simulink model "Test_N7"  (R2020b)
settings: Solver=ode3  StartTime=0.0  StopTime=inf  FixedStep=0.05  RelTol=1e-3
libraries: XBotBlockToolbox x2, Utilities x1

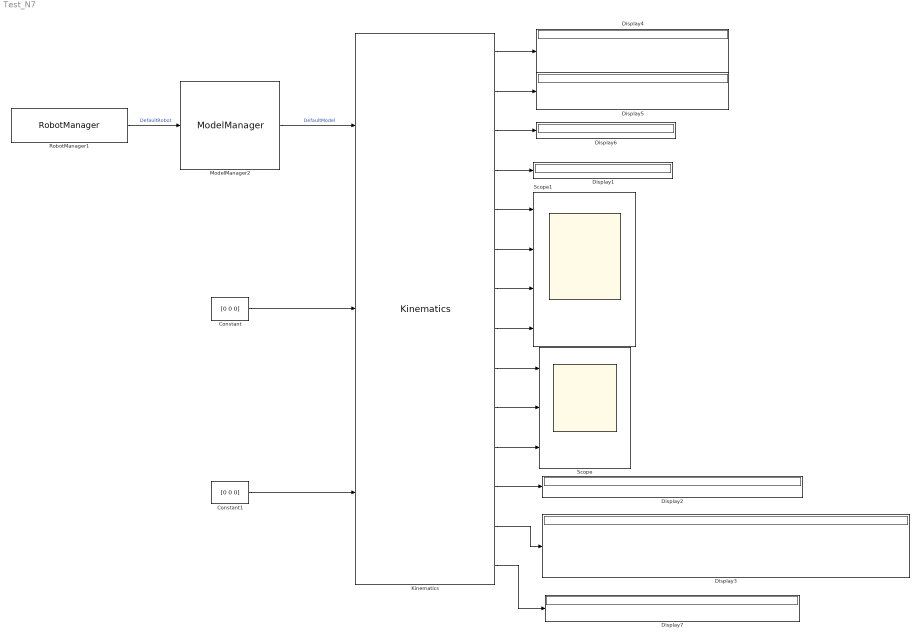
== system Test_N7 ==
  Constant : Constant  Value=[0 0 0]
  Constant1 : Constant  Value=[0 0 0]
  Display{1..7} (7 alike) : Display
  Kinematics : Utilities/Kinematics  ModelName=DefaultModel  PoseList={ 'Pose', 'RotMatrix', 'PointPos', 'PointAcc' }  SourceFrame=LWrMot3  LinkNamePose=LWrMot3  TwistList={ 'v_tw', 'a_tw', 'v_tw_rel', 'a_tw_rel' }  LinkName=LWrMot3  BaseLinkName=base_link  COMList={ 'p_COM', 'v_COM', 'a_COM', 'CM', 'CM_Matrix', 'CMMdotQdot' }
  ModelManager2 : XBotBlockToolbox/ModelManager  ModelName=DefaultModel  RobotName=DefaultRobot  UseExtModel=Off  SyncWithRobot=On  GetFloatingBaseList={}  SetFloatingBaseComponent=Off  GravityRequest=Off  ReadingsList={}  MechanicalLimitsList={}  MechanicalLimitsCheck=Off  MechanicalLimitsEnforce=Off  SensorList={}  ReferencesList={}  OldModelName=DefaultModel
  RobotManager1 : XBotBlockToolbox/RobotManager  RobotName=DefaultRobot  ModelName=DefaultModel  UseExtRobot=Off  SyncWithModel=Off  ReadingsList={}  MechanicalLimitsList={}  MechanicalLimitsCheck=Off  MechanicalLimitsEnforce=Off  SensorList={}  ReferencesList={}  OldRobotName=DefaultRobot
  Scope : Scope  NumInputPorts=3
  Scope1 : Scope  NumInputPorts=4
  wires:
  RobotManager1/1 -> ModelManager2/1  "DefaultRobot"
  ModelManager2/1 -> Kinematics/1  "DefaultModel"
  Kinematics/1 -> Display4/1
  Kinematics/2 -> Display5/1
  Kinematics/3 -> Display6/1
  Constant/1 -> Kinematics/2
  Kinematics/9 -> Scope/1
  Kinematics/10 -> Scope/2
  Kinematics/11 -> Scope/3
  Kinematics/5 -> Scope1/1
  Kinematics/6 -> Scope1/2
  Kinematics/7 -> Scope1/3
  Kinematics/8 -> Scope1/4
  Constant1/1 -> Kinematics/3
  Kinematics/4 -> Display1/1
  Kinematics/12 -> Display2/1
  Kinematics/13 -> Display3/1
  Kinematics/14 -> Display7/1
